simulink model "W03_F_windup"  (R2024b)
settings: Solver=ode4  StartTime=0  StopTime=T_final  FixedStep=h  RelTol=1e-3
values from neighbouring files (symbols this model uses):
  beta_c = 0    [W03_0_setup.m]
  k_neg = cfg.k_neg    [W03_0_setup.m]
  k_pos = cfg.k_pos    [W03_0_setup.m]
  Kd = 74.90    (= 74.9)    [W03_0_setup.m]
  Kp = 100.00    (= 100)    [W03_0_setup.m]
  mp = 25    [W03_0_setup.m]
  rp = [0.05 0 -0.35]'    [W03_0_setup.m]
  V_c = 0    [W03_0_setup.m]
  x0 = zeros(12,1)    [W03_0_setup.m]
undefined symbols (not defined in the file or in its folder): Kb, Ki, Nf, t_step, t_step2, u_step, u_step2, X_hi, X_lo
settings Model: Creator=admin  LastModifiedBy=admin
settings DataIOCC: ReturnWorkspaceOutputs=off

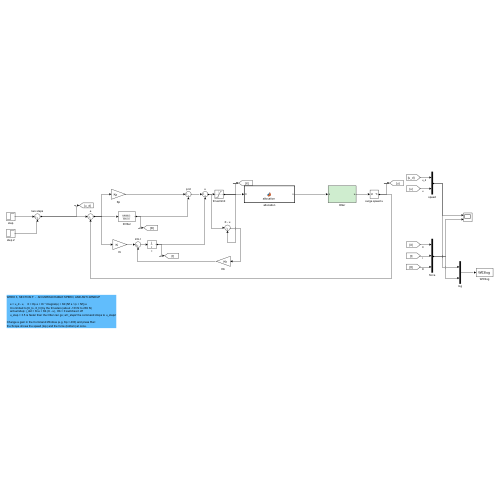
[thumbnail: Simulink's stored preview of the top-level diagram]
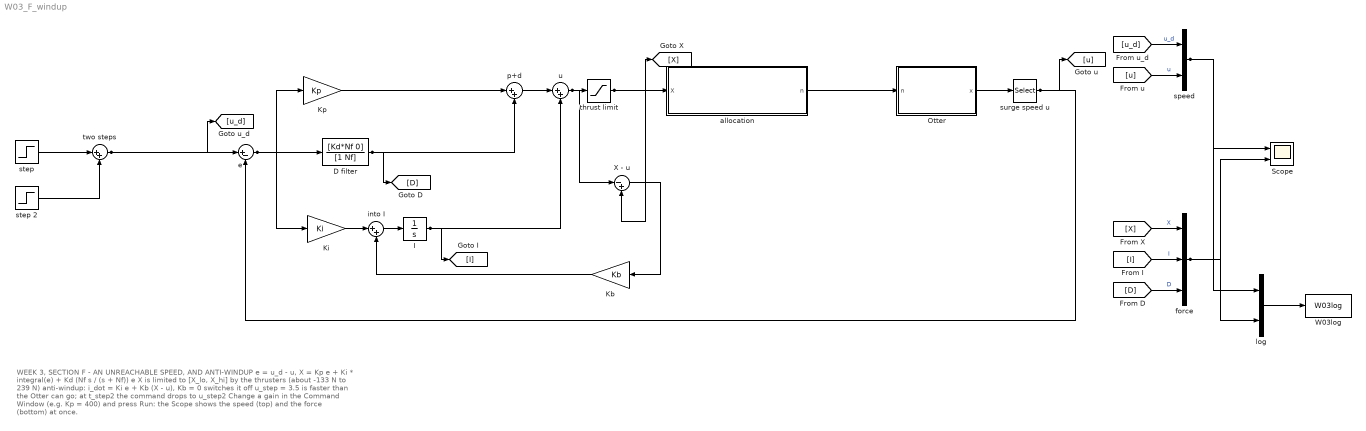
== system W03_F_windup ==
  note: WEEK 3, SECTION F  -  AN UNREACHABLE SPEED, AND ANTI-WINDUP
      |
      |     e = u_d - u,    X = Kp e + Ki * integral(e) + Kd (Nf s / (s + Nf)) e
      |     X is limited to [X_lo, X_hi] by the thrusters (about -133 N to 239 N)
      |     anti-windup: i_dot = Ki e + Kb (X - u),  Kb = 0 switches it off
      |     u_step = 3.5 is faster than the Otter can go; at t_step2 the command drops to u_step2
      |
      | Change a gain in the Command Window (e.g. Kp = 400) and press Run:
      | the Scope shows the speed (top) and the force (bottom) at once.
  D filter : TransferFcn  Numerator=[Kd*Nf 0]  Denominator=[1 Nf]
  I : Integrator
  Kb : Gain  Gain=Kb
  Ki : Gain  Gain=Ki
  Kp : Gain  Gain=Kp
  Otter : Subsystem
  Scope : Scope  NumInputPorts=2
  W03log : ToWorkspace  VariableName=W03log  SaveFormat=Structure With Time  SampleTime=-1
  X - u : Sum  Inputs=|-+
  allocation : MATLAB Function  TreatAsAtomicUnit=on
  e : Sum  Inputs=|+-
  force : Mux  Inputs=3
  into I : Sum  Inputs=|++
  log : Mux  Inputs=2
  p+d : Sum  Inputs=|++
  speed : Mux  Inputs=2
  step : Step  Time=t_step  After=u_step  SampleTime=0
  step 2 : Step  Time=t_step2  After=u_step2 - u_step  SampleTime=0
  surge speed u : Selector  InputPortWidth=12  IndexOptions=Index vector (dialog)  Indices=1  OutputSizes=1
  thrust limit : Saturate  UpperLimit=X_hi  LowerLimit=X_lo
  two steps : Sum  Inputs=|++
  u : Sum  Inputs=|++
  wires:
  step/1 -> two steps/1
  step 2/1 -> two steps/2
  two steps/1 -> e/1, [u_d]
  e/1 -> Kp/1, D filter/1, Ki/1
  Kp/1 -> p+d/1
  D filter/1 -> p+d/2, [D]
  Ki/1 -> into I/1
  into I/1 -> I/1
  p+d/1 -> u/1
  I/1 -> u/2, [I]
  u/1 -> thrust limit/1, X - u/1
  thrust limit/1 -> X - u/2, [X], allocation/1(X)
  X - u/1 -> Kb/1
  Kb/1 -> into I/2
  allocation/1(n) -> Otter/1(n)
  Otter/1(x) -> surge speed u/1
  surge speed u/1 -> [u], e/2
  [u_d] -> speed/1  "u_d"
  [u] -> speed/2  "u"
  [X] -> force/1  "X"
  [I] -> force/2  "I"
  [D] -> force/3  "D"
  speed/1 -> Scope/1, log/1
  force/1 -> Scope/2, log/2
  log/1 -> W03log/1

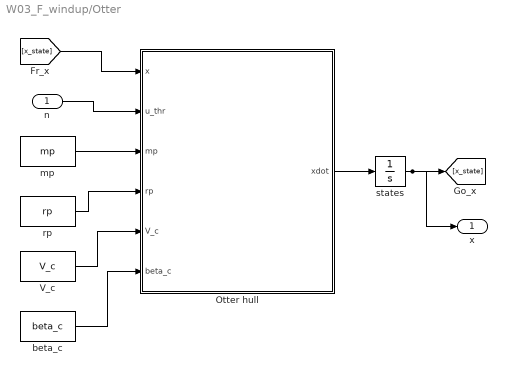
== system W03_F_windup/Otter ==
  n : Inport
  Otter hull : MATLAB Function  TreatAsAtomicUnit=on
  V_c : Constant  Value=V_c
  beta_c : Constant  Value=beta_c
  mp : Constant  Value=mp
  rp : Constant  Value=rp
  states : Integrator  InitialCondition=x0
  x : Outport
  wires:
  [x_state] -> Otter hull/1(x)
  n/1 -> Otter hull/2(u_thr)
  mp/1 -> Otter hull/3(mp)
  Otter hull/1(xdot) -> states/1
  beta_c/1 -> Otter hull/6(beta_c)
  rp/1 -> Otter hull/4(rp)
  V_c/1 -> Otter hull/5(V_c)
  states/1 -> [x_state], x/1

== matlab function W03_F_windup/Otter/Otter hull ==
  data: x input; xdot output double size=[12 1]; u_thr input; mp input; rp input; V_c input; beta_c input
function xdot = otter_hull(x, u_thr, mp, rp, V_c, beta_c)
% Fossen's otter.m, called unchanged from Tools/MSS/VESSELS.
%
%   x       12 states, fed back from the integrator
%   u_thr   propeller shaft speeds [rad/s]
%
% otter.m is not written for code generation, so the call is extrinsic and
% xdot has to be pre-sized for Simulink to know the output width.
coder.extrinsic('otter');

xdot = zeros(12,1);
xdot = otter(x, u_thr, mp, rp, V_c, beta_c);
end

== matlab function W03_F_windup/allocation ==
  data: X input; n output double size=[2 1]; k_pos parameter; k_neg parameter
function n = allocation(X, k_pos, k_neg)
%#codegen
%ALLOCATION  전진력 X [N] 를 두 프로펠러의 축 회전수 n [rad/s] 로 바꾼다.
%            Turn the surge force X [N] into the shaft speeds n [rad/s] of the two propellers.
%
%   k_pos, k_neg 는 작업공간 변수 (W03_0_setup) 에서 온다 — 블록의 포트가 아니다.
%   k_pos and k_neg come from the workspace (W03_0_setup), not from ports.

% 1) 똑바로 갈 때 두 프로펠러는 같은 일을 한다: 각자 X 의 절반.
%    Going straight, both propellers do the same work: half of X each.
T = X/2;

% 2) 프로펠러 곡선 T = k n|n| (1주차) 을 n 에 대해 푼다.
%    앞으로 밀 때와 뒤로 당길 때 계수가 다르다 (k_pos > k_neg).
%    Solve the propeller curve T = k n|n| (Week 1) for n; the coefficient
%    differs ahead and astern (k_pos > k_neg).
if T >= 0
    n1 =  sqrt( T / k_pos);      % 앞으로 / ahead
else
    n1 = -sqrt(-T / k_neg);      % 뒤로 / astern
end

% 3) 두 축에 같은 회전수. Otter 는 [좌현; 우현] 순서로 받는다.
%    The same speed on both shafts; the Otter takes [port; starboard].
n = [n1; n1];
end
